simulink model "sf_superstep"  (Simulink 7.6)
settings: Solver=FixedStepDiscrete  StartTime=0.0  StopTime=10.0  FixedStep=1  RelTol=1e-3
settings Model: Creator=The MathWorks Inc.  ExtModeAutoUpdateStatusClock=off
settings SolverCC: InsertRTBMode=Auto
settings OptimizationCC: InitFltsAndDblsToZero=on
settings DebuggingCC: SolverPrmCheckMsg=none  StrictBusMsg=Warning
settings SFSimCC: SimParseCustomCode=off

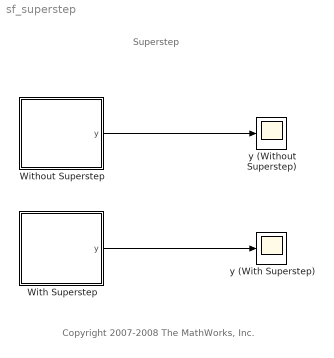
== system sf_superstep ==
  note: Superstep
  note: Copyright 2007-2008 The MathWorks, Inc.
  With Superstep : Stateflow chart  TreatAsAtomicUnit=on
  Without Superstep : Stateflow chart  TreatAsAtomicUnit=on
  y (With Superstep) : Scope
  "y (Without Superstep) " : Scope
  wires:
  Without Superstep/1(y) -> "y (Without Superstep) "/1
  With Superstep/1(y) -> y (With Superstep)/1

== stateflow chart Without Superstep ==
  state A
    en: y = 1;
  state B
    en: y = 2;
  state C
    en: y = 3;
  A -> B
  B -> C : [ x == 1 ]
  (default) -> A : { x = 1; }
  data: y output double; x local double

== stateflow chart With Superstep ==
  settings: enableNonTerminalStates=1
  state A
    en: y = 1;
  state B
    en: y = 2;
  state C
    en: y = 3;
  A -> B
  B -> C : [ x == 1 ]
  (default) -> A : { x = 1; }
  data: y output double; x local double
